simulink model "disturbo_d"  (R2022b)
settings: Solver=VariableStepAuto  StartTime=0.0  StopTime=10.0  RelTol=1e-3
model workspace (MAT data in the model file):
  amplitude_d = Simulink.Parameter
  amplitude_d.Value = 1
  amplitude_d.DataType = 'auto'
  amplitude_d.Complexity = 'real'
  amplitude_d.Dimensions = [1 1]
settings Model: ParameterArgumentNames=amplitude_d  Creator=eleon  LastModifiedBy=eleon

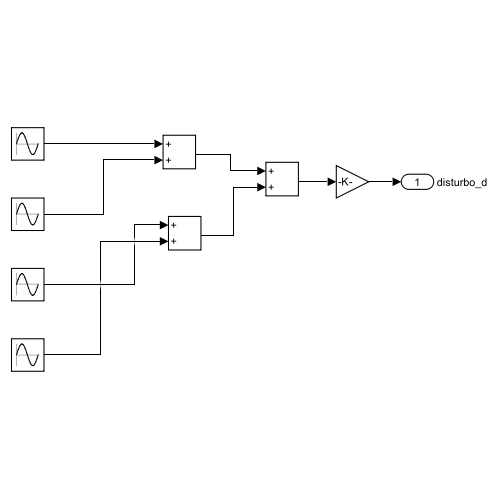
[thumbnail: Simulink's stored preview of the top-level diagram]
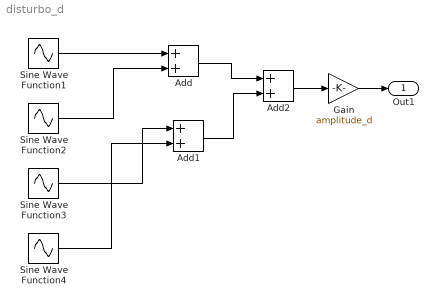
== system disturbo_d ==
  Add : Sum
  Add1 : Sum
  Add2 : Sum
  Gain : Gain  Gain=amplitude_d
  Sine Wave Function1 : Sin  Amplitude=0.1  Frequency=0.025  SampleTime=0
  Sine Wave Function2 : Sin  Amplitude=0.1  Frequency=0.025*2  SampleTime=0
  Sine Wave Function3 : Sin  Amplitude=0.1  Frequency=0.025*3  SampleTime=0
  Sine Wave Function4 : Sin  Amplitude=0.1  Frequency=0.025*4  SampleTime=0
  Out1 : Outport  SignalName=disturbo_d
  wires:
  Add/1 -> Add2/1
  Add1/1 -> Add2/2
  Sine Wave Function4/1 -> Add1/2
  Sine Wave Function3/1 -> Add1/1
  Sine Wave Function2/1 -> Add/2
  Sine Wave Function1/1 -> Add/1
  Add2/1 -> Gain/1
  Gain/1 -> Out1/1
